simulink model "test04"  (R2025b)
settings: Solver=VariableStepAuto  StartTime=0.0  StopTime=60  RelTol=1e-3
settings Model: Creator=sanborkl  LastModifiedBy=sanborkl

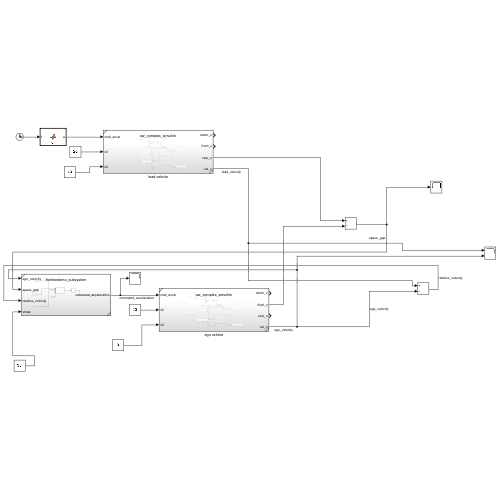
[thumbnail: Simulink's stored preview of the top-level diagram]
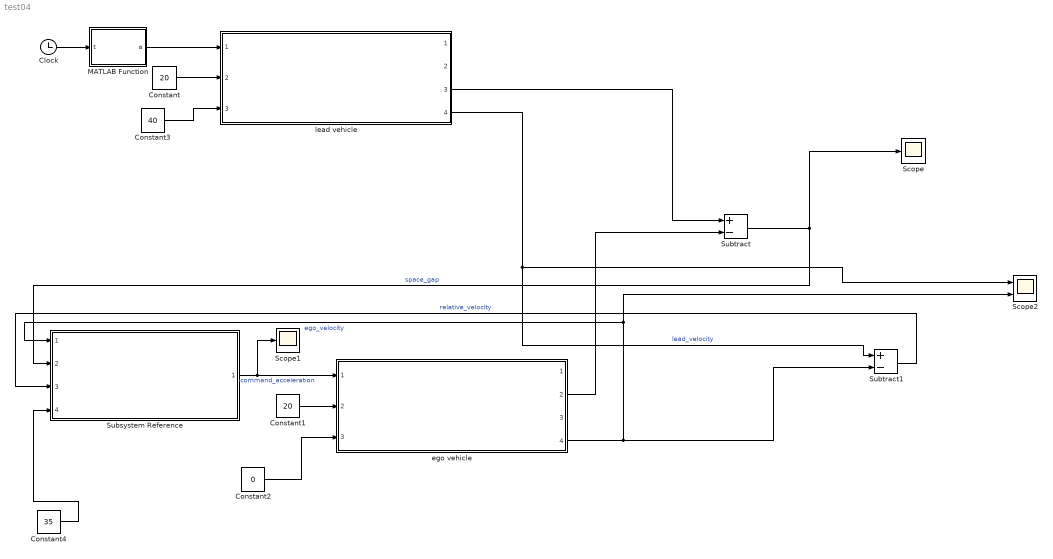
== system test04 ==
  Clock : Clock
  Constant : Constant  Value=20
  Constant1 : Constant  Value=20
  Constant2 : Constant  Value=0
  Constant3 : Constant  Value=40
  Constant4 : Constant  Value=35
  MATLAB Function : MATLAB Function  TreatAsAtomicUnit=on
  Scope : Scope
      settings: ActiveDisplayYMinimum=3.3198341313451163  ActiveDisplayYMaximum=70.12438332925575
  Scope1 : Scope
      settings: ActiveDisplayYMinimum=-3.4401005593365008  ActiveDisplayYMaximum=0.96090503402850735
  Scope2 : Scope  NumInputPorts=2
      settings: ActiveDisplayYMinimum=-2.4999999999999996  ActiveDisplayYMaximum=22.5  DataLoggingVariableName=ScopeData2
  Subsystem Reference : Subsystem  ReferencedSubsystem=frontierdemo_subsystem
  Subtract : Sum  Inputs=+-
  Subtract1 : Sum  Inputs=+-
  ego vehicle : Subsystem  ReferencedSubsystem=car_complex_simulink
  lead vehicle : Subsystem  ReferencedSubsystem=car_complex_simulink
  wires:
  Subsystem Reference/1 -> Scope1/1, ego vehicle/1  "command_acceleration"
  Subtract/1 -> Subsystem Reference/2, Scope/1  "space_gap"
  Constant1/1 -> ego vehicle/2
  Constant/1 -> lead vehicle/2
  lead vehicle/3 -> Subtract/1
  Subtract1/1 -> Subsystem Reference/3  "relative_velocity"
  lead vehicle/4 -> Scope2/1, Subtract1/1  "lead_velocity"
  Constant2/1 -> ego vehicle/3
  ego vehicle/2 -> Subtract/2
  Constant3/1 -> lead vehicle/3
  Clock/1 -> MATLAB Function/1(t)
  MATLAB Function/1(a) -> lead vehicle/1
  ego vehicle/4 -> Scope2/2, Subsystem Reference/1, Subtract1/2  "ego_velocity"
  Constant4/1 -> Subsystem Reference/4

== matlab function test04/MATLAB Function ==
  data: t input; a output
function a = fcn(t)

a = 0;

if t > 10
    a = -4.5;
end
